simulink model "GripTask"  (R2022b)
settings: Solver=FixedStepDiscrete  StartTime=0.0  StopTime=Inf  FixedStep=0.001  RelTol=1e-3  EnableMultiTasking=on
InitFcn:
  | parambus = Simulink.Bus;
  | idx = 0;
  | 
  | idx = idx + 1;
  | parambus.Elements(idx) = Simulink.BusElement;
  | parambus.Elements(idx).Name = 'ScreenOn';
  | parambus.Elements(idx).DataType = 'uint8';
  | parambus.Elements(idx).Dimensions = [1, 1];
  | 
  | idx = idx + 1;
  | parambus.Elements(idx) = Simulink.BusElement;
  | parambus.Elements(idx).Name = 'DelayPeriod';
  | parambus.Elements(idx).DataType = 'uint16';
  | parambus.Elements(idx).Dimensions = [1, 2];
  | 
  | idx = idx + 1;
  | parambus.Elements(idx) = Simulink.BusElement;
  | parambus.Elements(idx).Name = 'TargetHoldTime';
  | parambus.Elements(idx).DataType = 'uint16';
  | parambus.Elements(idx).Dimensions = [1, 1];
  | 
  | idx = idx + 1;
  | parambus.Elements(idx) = Simulink.BusElement;
  | parambus.Elements(idx).Name = 'TargetScaling';
  | parambus.Elements(idx).DataType = 'uint8';
  | parambus.Elements(idx).Dimensions = [1, 1];
  | 
  | idx = idx + 1;
  | parambus.Elements(idx) = Simulink.BusElement;
  | parambus.Elements(idx).Name = 'TrialTimeout';
  | parambus.Elements(idx).DataType = 'uint16';
  | parambus.Elements(idx).Dimensions = [1, 1];
  | 
  | idx = idx + 1;
  | parambus.Elements(idx) = Simulink.BusElement;
  | parambus.Elements(idx).Name = 'GripCalibration';
  | parambus.Elements(idx).DataType = 'single';
  | parambus.Elements(idx).Dimensions = [1, 2];
  | 
  | idx = idx + 1;
  | parambus.Elements(idx) = Simulink.BusElement;
  | parambus.Elements(idx).Name = 'GripTarget';
  | parambus.Elements(idx).DataType = 'single';
  | parambus.Elements(idx).Dimensions = [1, 1];
  | 
  | idx = idx + 1;
  | parambus.Elements(idx) = Simulink.BusElement;
  | parambus.Elements(idx).Name = 'TaskMode';
  | parambus.Elements(idx).DataType = 'uint8';
  | parambus.Elements(idx).Dimensions = [1, 1];
  | 
  | idx = idx + 1;
  | parambus.Elements(idx) = Simulink.BusElement;
  | parambus.Elements(idx).Name = 'BuzzDuration';
  | parambus.Elements(idx).DataType = 'uint16';
  | parambus.Elements(idx).Dimensions = [1, 1];
  | 
  | FileLoggerEntry = Simulink.Bus;
  | FileLoggerEntry.Elements(1) = Simulink.BusElement;
  | FileLoggerEntry.Elements(1).Name = 'FileType';
  | FileLoggerEntry.Elements(1).DataType = 'uint8';
  | FileLoggerEntry.Elements(1).Dimensions = [1, 1];
  | FileLoggerEntry.Elements(2) = Simulink.BusElement;
  | FileLoggerEntry.Elements(2).Name = 'FieldName';
  | FileLoggerEntry.Elements(2).DataType = 'uint8';
  | FileLoggerEntry.Elements(2).Dimensions = [1, 20];
  | FileLoggerEntry.Elements(3) = Simulink.BusElement;
  | FileLoggerEntry.Elements(3).Name = 'DataType';
  | FileLoggerEntry.Elements(3).DataType = 'uint8';
  | FileLoggerEntry.Elements(3).Dimensions = [1, 6];
  | FileLoggerEntry.Elements(4) = Simulink.BusElement;
  | FileLoggerEntry.Elements(4).Name = 'NumElements';
  | FileLoggerEntry.Elements(4).DataType = 'uint8';
  | FileLoggerEntry.Elements(4).Dimensions = [1, 1];
  | FileLoggerEntry.Elements(5) = Simulink.BusElement;
  | FileLoggerEntry.Elements(5).Name = 'Data';
  | FileLoggerEntry.Elements(5).DataType = 'double';
  | FileLoggerEntry.Elements(5).Dimensions = [1, 255];
undefined symbols (not defined in the file): Ended, Single
libraries: speedgoatlib_IO191 x3, Lab_Library x2, slrealtimeseriallib x1, slrealtimeiplib x1
settings Model: Creator=irwin  LastModifiedBy=l-zirwin
settings SolverCC: ConcurrentTasks=on  AlgebraicLoopSolver=TrustRegion  PositivePriorityOrder=on  InsertRTBMode=Never (minimum delay)
settings DataIOCC: SaveFormat=Array  SaveState=on  SignalLoggingName=logsOut
settings OptimizationCC: BlockReduction=off  BooleanDataType=off  OptimizeBlockIOStorage=off  BufferReuse=off  GlobalBufferReuse=off  ExpressionFolding=off  LocalBlockOutputs=off  InitFltsAndDblsToZero=on  OptimizeDataStoreBuffers=off  BusAssignmentInplaceUpdate=off
settings DebuggingCC: SaveWithParameterizedLinksMsg=none  UnderspecifiedInitializationDetection=Classic  MergeDetectMultiDrivingBlocksExec=none  CheckExecutionContextPreStartOutputMsg=on  SignalResolutionControl=TryResolveAllWithWarning  TasksWithSamePriorityMsg=none  UnconnectedInputMsg=warning  UnconnectedOutputMsg=warning  UnconnectedLineMsg=warning  SFUnexpectedBacktrackingDiag=warning  SFNoUnconditionalDefaultTransitionDiag=warning  SFExecutionAtInitializationDiag=none  SFMachineParentedDataDiag=warning  ArithmeticOperatorsInVariantConditions=warning
settings HardwareCC: ProdBitPerLong=64  ProdLongLongMode=on  ProdHWDeviceType=Intel->x86-64 (Linux 64)
settings ModelReferenceCC: EnableRefExpFcnMdlSchedulingChecks=on  PropagateSignalLabelsOutOfModel=off
settings SFSimCC: SimUseLocalCustomCode=off  SimTargetLang=C++
settings RTWCC: Description=Simulink Real-Time  SystemTargetFile=slrealtime.tlc  TemplateMakefile=slrealtime_default_tmf  RTWUseLocalCustomCode=off  Toolchain=Simulink Real-Time Toolchain  BuildConfiguration=Faster Runs  CodeExecutionProfiling=on  TargetLang=C++  DLArmComputeVersion=19.05
settings CodeAppCC: StateflowObjectComments=on
settings SimulinkRealTimeTargetCC: MATLABClassNameForMDSCustomization=Simulink.SoftwareTarget.GRTCustomization  UseGCCFastMath=on
settings ConfigComp: CovMetricSettings=dw  CovSaveCumulativeToWorkspaceVar=on  CovSaveSingleToWorkspaceVar=on  CovExternalEMLEnable=off  CovSFcnEnable=off

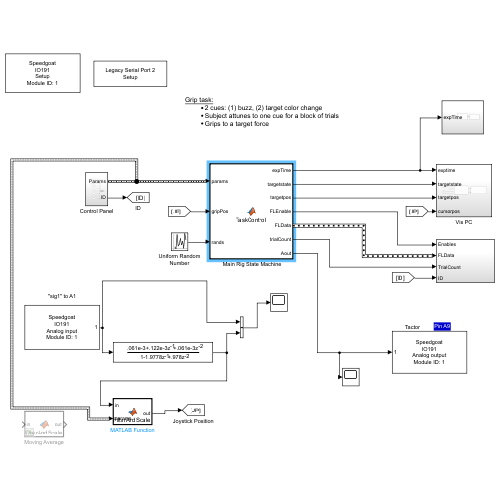
[thumbnail: Simulink's stored preview of the top-level diagram]
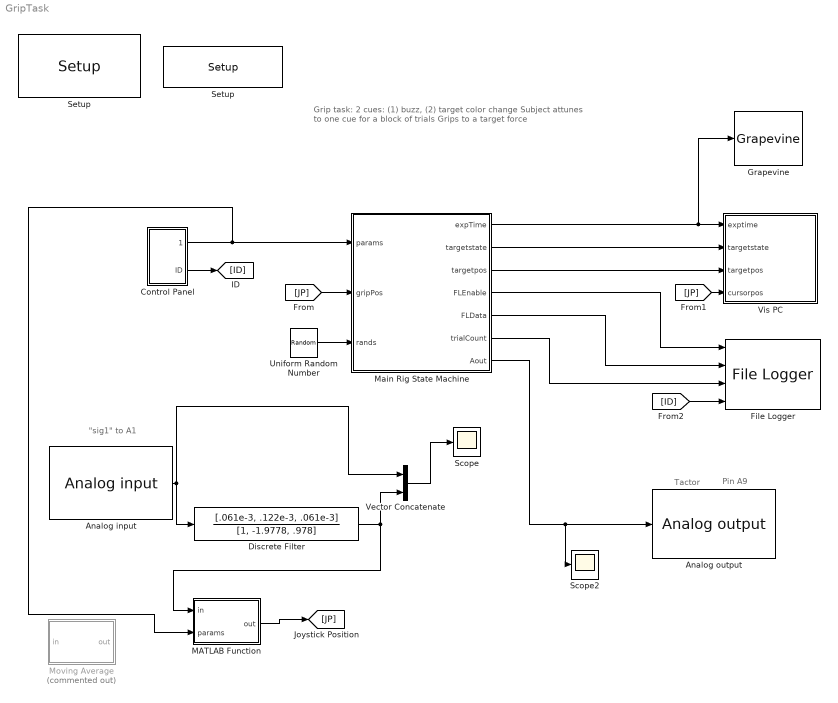
== system GripTask ==
  note: "sig1" to A1
  note: Grip task:
      | 2 cues: (1) buzz, (2) target color change
      | Subject attunes to one cue for a block of trials
      | Grips to a target force
  note: Tactor
  note: Pin A9
  " Main Rig State Machine" : MATLAB Function  TreatAsAtomicUnit=on
  "Analog input " : speedgoatlib_IO191/Analog input   parModuleId=1  parSampleTime=-1  parPciSlot=-1  parAdcChannels=1  parAdcMode=2  parAdcRanges=4  parAdcRate=100000  parAdcInitValues=[0 0]  parAdcResets=[1 1]
      settings: SourceProductName=Simulink Real-Time: Speedgoat I/O Blockset
  "Analog output " : speedgoatlib_IO191/Analog output   parModuleId=1  parSampleTime=-1  parPciSlot=-1  parDacChannels=1  parModuleType=1  parDacRanges=5  parDacInitValues=0  parDacResets=1
      settings: SourceProductName=Simulink Real-Time: Speedgoat I/O Blockset
  Control Panel : Subsystem
  Discrete Filter : DiscreteFilter  Numerator=[.061e-3, .122e-3, .061e-3]  Denominator=[1, -1.9778, .978]
  File Logger : Lab_Library/File Logger  SystemSampleTime=-1  VariantActivationTime=update diagram  Latency=0  AutoFrameSizeCalculation=off
  Grapevine : Lab_Library/Grapevine  SystemSampleTime=-1  VariantActivationTime=update diagram  Latency=0  AutoFrameSizeCalculation=off
  MATLAB Function : MATLAB Function  TreatAsAtomicUnit=on
  Moving Average : MATLAB Function  Commented=on  TreatAsAtomicUnit=on
  Scope : Scope
  Scope2 : Scope
  Setup : slrealtimeseriallib/Mainboard/Setup  port=Legacy Serial Port 2  baud=115200  width=8  nstop=1  parity=None  ctsmode=off
  "Setup " : speedgoatlib_IO191/Setup   parModuleId=1  parPciSlot=-1  parTriggerSignal=TTL  parAdcChannels=1  parAdcRanges=4  parAdcChannel1=on  parAdcChannel2=off  parAdcChannel3=off  parAdcChannel4=off  parAdcChannel5=off  parAdcChannel6=off  parAdcChannel7=off  parAdcChannel8=off  parAdcMode=Single-Ended  parAdcRate=100000  parAdcRange11=+-5.12 V  parAdcRange21=+-24.576 V  parAdcRange12=+-2.56 V  parAdcRange22=+-24.576 V  parAdcRange13=+-2.56 V  parAdcRange23=+-24.576 V  parAdcRange14=+-2.56 V  parAdcRange24=+-24.576 V  parAdcRange15=+-10.24 V  parAdcRange25=+-24.576 V  parAdcRange16=+-10.24 V  parAdcRange26=+-24.576 V  parAdcRange17=+-10.24 V  parAdcRange27=+-24.576 V  parAdcRange18=+-10.24 V  parAdcRange28=+-24.576 V  parDacChannels=1  parDacChannel1=on  parDacChannel2=off  parDacChannel3=off  parDacChannel4=off  parDacMode=Single-Ended  parDacRanges=5  parDacInitValues=0  parDacResets=1  parDacRange1=+-2.5 V  parDacInitValue1=0  parDacReset1=on  parDacRange2=+-10 V  parDacInitValue2=0  parDacReset2=on  parDacRange3=+-10 V  parDacInitValue3=0  parDacReset3=on  parDacRange4=+-10 V  parDacInitValue4=0  parDacReset4=on  parDiChannels=[1 2 3 4 5 6 7 8 9 10 11 12 13 14 15 16]  parDoChannels=zeros(1,0)  parDioFirstControl=zeros(1,0)  parDioSecondControl=0  parDioChannel1=In  parExtra1=I  parExtra2=I  parExtra3=I  parDioChannel2=In  parDioChannel3=In  parDioChannel4=In  parDioChannel5=In  parDioChannel6=In  parDioChannel7=In  parDioChannel8=In  parDioChannel9=In  parDoInitValues=[0 0 0 0]  parDoResets=[1 1 1 1]  parDoInitValue1=0  parDoReset1=on  parDoInitValue2=0  parDoReset2=on  parDoInitValue3=0  parDoReset3=on  parDoInitValue4=0  parDoReset4=on  parDoInitValue5=0  parDoReset5=on  parDoInitValue6=0  parDoReset6=on  parDoInitValue7=0  parDoReset7=on  parDoInitValue8=0  parDoReset8=on  parDoInitValue9=0  parDoReset9=on  parDoInitValue10=0  parDoReset10=on  parDoInitValue11=0  parDoReset11=on  parDoInitValue12=0  parDoReset12=on  parDoInitValue13=0  parDoReset13=on  parDoInitValue14=0  parDoReset14=on  parDoInitValue15=0  parDoReset15=on  parDoInitValue16=0  parDoReset16=on
      settings: SourceProductName=Simulink Real-Time: Speedgoat I/O Blockset
  Uniform Random Number : UniformRandomNumber  Minimum=[0, 0, 0, 0]  Maximum=[2, 2, 2, 1]  Seed=[0, 64, 71, 6]  SampleTime=.001
  Vector Concatenate : Concatenate
  Vis PC : Subsystem
  wires:
  " Main Rig State Machine"/1(expTime) -> Grapevine/1, Vis PC/1(exptime)
  " Main Rig State Machine"/2(targetstate) -> Vis PC/2(targetstate)
  " Main Rig State Machine"/4(FLEnable) -> File Logger/1
  " Main Rig State Machine"/5(FLData) -> File Logger/2
  " Main Rig State Machine"/6(trialCount) -> File Logger/3
  [JP] -> " Main Rig State Machine"/2(gripPos)
  [JP] -> Vis PC/4(cursorpos)
  Control Panel/2(ID) -> [ID]
  [ID] -> File Logger/4
  Control Panel/1(Params) -> MATLAB Function/2(params), " Main Rig State Machine"/1(params)
  Uniform Random Number/1 -> " Main Rig State Machine"/3(rands)
  " Main Rig State Machine"/3(targetpos) -> Vis PC/3(targetpos)
  "Analog input "/1 -> Vector Concatenate/1, Discrete Filter/1
  " Main Rig State Machine"/7(Aout) -> Scope2/1, "Analog output "/1
  Discrete Filter/1 -> MATLAB Function/1(in), Vector Concatenate/2
  Vector Concatenate/1 -> Scope/1
  MATLAB Function/1(out) -> [JP]

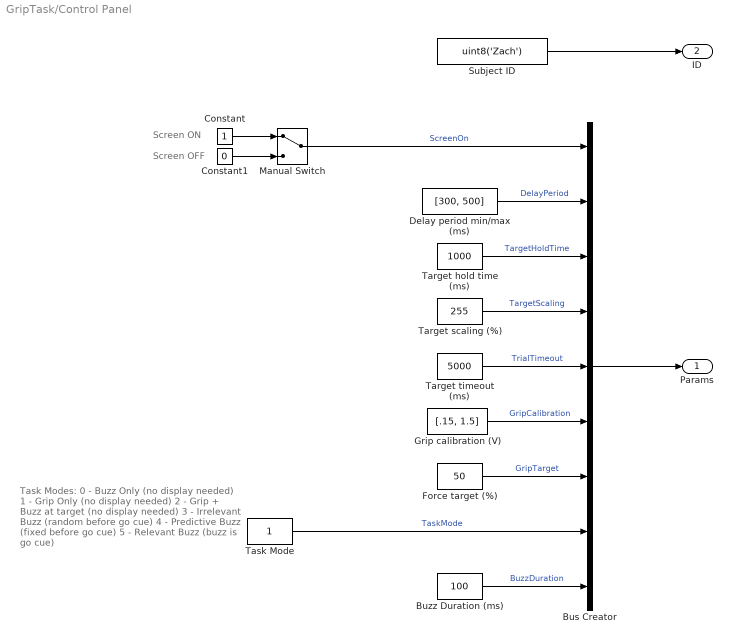
== system GripTask/Control Panel ==
  note: Task Modes:
      | 0 - Buzz Only (no display needed)
      | 1 - Grip Only (no display needed)
      | 2 - Grip + Buzz at target (no display needed)
      | 3 - Irrelevant Buzz (random before go cue)
      | 4 - Predictive Buzz (fixed before go cue)
      | 5 - Relevant Buzz (buzz is go cue)
  note: Screen ON
  note: Screen OFF
  Bus Creator : BusCreator  Inputs=9  OutDataTypeStr=Bus: parambus  NonVirtualBus=on
      settings: InheritFromInputs=off
  Buzz Duration (ms) : Constant  Value=100  OutDataTypeStr=uint16
  Constant : Constant  OutDataTypeStr=uint8
  Constant1 : Constant  Value=0  OutDataTypeStr=uint8
  Delay period min/max (ms) : Constant  Value=[300, 500]  OutDataTypeStr=uint16
  Force target (%) : Constant  Value=50  OutDataTypeStr=single
  Grip calibration (V) : Constant  Value=[.15, 1.5]  OutDataTypeStr=single
  Manual Switch : ManualSwitch
  Subject ID : Constant  Value=uint8('Zach')  OutDataTypeStr=uint8
  Target hold time (ms) : Constant  Value=1000  OutDataTypeStr=uint16
  Target scaling (%) : Constant  Value=255  OutDataTypeStr=uint8
  Target timeout (ms) : Constant  Value=5000  OutDataTypeStr=uint16
  Task Mode : Constant  OutDataTypeStr=uint8
  Params : Outport
  ID : Outport  Port=2
  wires:
  Delay period min/max (ms)/1 -> Bus Creator/2  "DelayPeriod"
  Manual Switch/1 -> Bus Creator/1  "ScreenOn"
  Constant1/1 -> Manual Switch/2
  Constant/1 -> Manual Switch/1
  Bus Creator/1 -> Params/1
  Target hold time (ms)/1 -> Bus Creator/3  "TargetHoldTime"
  Subject ID/1 -> ID/1
  Target timeout (ms)/1 -> Bus Creator/5  "TrialTimeout"
  Target scaling (%)/1 -> Bus Creator/4  "TargetScaling"
  Grip calibration (V)/1 -> Bus Creator/6  "GripCalibration"
  Force target (%)/1 -> Bus Creator/7  "GripTarget"
  Task Mode/1 -> Bus Creator/8  "TaskMode"
  Buzz Duration (ms)/1 -> Bus Creator/9  "BuzzDuration"

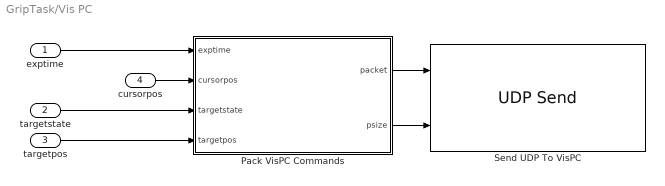
== system GripTask/Vis PC ==
  exptime : Inport
  targetstate : Inport  Port=2
  targetpos : Inport  Port=3
  cursorpos : Inport  Port=4
  Pack VisPC Commands : MATLAB Function  TreatAsAtomicUnit=on
  Send UDP To VisPC : slrealtimeiplib/UDP Send  useHostTargetConn=off  toAddress='192.168.44.2'  toPort=11114  sampleTime=-1  enableMessage=off  ipAddress='192.168.44.1'  localPort=11114
  wires:
  cursorpos/1 -> Pack VisPC Commands/2(cursorpos)
  Pack VisPC Commands/1(packet) -> Send UDP To VisPC/1
  Pack VisPC Commands/2(psize) -> Send UDP To VisPC/2
  targetstate/1 -> Pack VisPC Commands/3(targetstate)
  exptime/1 -> Pack VisPC Commands/1(exptime)
  targetpos/1 -> Pack VisPC Commands/4(targetpos)

== matlab function GripTask/Vis PC/Pack VisPC Commands ==
  data: exptime input; cursorpos input; targetstate input; packet output; psize output; targetpos input
%
% targetstate [4 x 3]: state of each target (home, narrow, wide)
%   * Row 1: Target visibility
%   * Row 2: Target hit indicators
%   * Row 3: Target sizes
%   * Row 4: Target fill indicator

% targetpos [3 x 2]: x/y position of each target (home, narrow, wide)
%   * Col 1: Left position
%   * Col 2: Top position

function [packet, psize] = CreateVisPacket(exptime, cursorpos, targetstate, targetpos)

persistent position scale color visibility fill ...
           hitcolor basecolor ...
           hometarget reachtarget_narrow reachtarget_wide cursor

if (isempty(position))

    % definitions for available objects:
    hometarget = uint8(1);
    reachtarget_narrow = uint8(2);
    reachtarget_wide = uint8(3);
    cursor = uint8(4);
    
    % definitions for available object properties:
    position = uint8(1);
    visibility = uint8(2);
    color = uint8(3);
    scale = uint8(4);
    fill = uint8(5);

    % default property values:
    hitcolor = uint8([0, 0, 255]);
    basecolor = uint8([255, 0, 0]);

end

%%% Packet structure:
%%% [experiment_time(4b), [object_id(1b), property_id(1b), property_value(xb)] ...]

% Visibility:
pvisible = [hometarget, visibility, targetstate(1,hometarget), ...
            reachtarget_narrow, visibility, targetstate(1,reachtarget_narrow), ...
            reachtarget_wide, visibility, targetstate(1,reachtarget_wide), ...
            cursor, visibility, any(targetstate(1,:))]; % cursor visible if any target is also visible, otherwise not


% Scaling:
pscaling = [hometarget, scale, targetstate(3,hometarget), ...
            reachtarget_narrow, scale, targetstate(3,reachtarget_narrow), ...
            reachtarget_wide, scale, targetstate(3,reachtarget_wide)];


% Color:
pcolor = [];
if (targetstate(2,hometarget))
    pcolor = [pcolor, hometarget, color, hitcolor];
else
    pcolor = [pcolor, hometarget, color, basecolor];
end
if (targetstate(2,reachtarget_narrow))
    pcolor = [pcolor, reachtarget_narrow, color, hitcolor];
else
    pcolor = [pcolor, reachtarget_narrow, color, basecolor];
end
if (targetstate(2,reachtarget_wide))
    pcolor = [pcolor, reachtarget_wide, color, hitcolor];
else
    pcolor = [pcolor, reachtarget_wide, color, basecolor];
end


% Fill:
pfill = [hometarget, fill, targetstate(4,hometarget), ...
            reachtarget_narrow, fill, targetstate(4,reachtarget_narrow), ...
            reachtarget_wide, fill, targetstate(4,reachtarget_wide)];


% Position:
pposition = [cursor, position, typecast([uint16(800), cursorpos], 'uint8'), ...
             hometarget, position, typecast(uint16(targetpos(hometarget,:)), 'uint8'), ...
             reachtarget_narrow, position, typecast(uint16(targetpos(reachtarget_narrow,:)), 'uint8'), ...
             reachtarget_wide, position, typecast(uint16(targetpos(reachtarget_wide,:)), 'uint8')];


% Collect into single packet, compute size, then pad to final size:
temppacket = [typecast(exptime, 'uint8'), pvisible, pscaling, pcolor, pfill, pposition];
psize = length(temppacket);
packet = [temppacket, zeros(1,1500 - psize, 'uint8')];

== matlab function GripTask/ Main Rig State Machine ==
  data: expTime output uint32 size=1; params input; gripPos input; rands input; targetstate output; targetpos output; FLEnable output; FLData output Bus: FileLoggerEntry; trialCount output; Aout output double size=1
function [expTime, targetstate, targetpos, FLEnable, FLData, trialCount, Aout] = TaskControl(params, gripPos, rands)

persistent exp_state trial_state exp_time trial_time trial_count intparams extparams...
           targpos prev_time FLStruct

if (isempty(exp_state))
    exp_state = uint8(0);           % Experiment state variable
    trial_state = uint8(0);         % Trial state variable
    exp_time = uint32(0);           % Current experiment time
    trial_time = uint32(0);         % Current trial time
    trial_count = uint16(0);        % Count of the trials in the current run
    extparams = params;             % Initialize parameters to incoming struct
    prev_time = double(-1);         % Marker for timing
    FLStruct = genFLStruct();       % Struct array for File Logger data

    intparams = struct('TaskMode', uint8(0), ...           % 6 different task modes
                       'DelayTime', uint16(0), ...          % delay period (ms)
                       'TrialSuccess', uint8(0), ...        % trial success indicator
                       'BlankTrial', uint8(0), ...          % indicator that screen was turned off
                       'TargetHit', zeros(1,3,'uint8'), ... % hit indicators for each target + home
                       'TargetFill', ones(1,3,'uint8'), ... % fill indicators for each target + home
                       'TargetVis', zeros(1,3,'uint8'), ...  % visbility indicators for each target + home
                       'BuzzDuration', uint16(0), ...      % Duration of buzz pulse
                       'PerturbDir', single(0));            % direction of perturbation for each trial

end

%%%%%%%%%%%%%%%%%%%%%%%%%%%%%%% Defines %%%%%%%%%%%%%%%%%%%%%%%%%%%%%%%%%%%

% Trial states:
tstate = struct('INIT',  uint8(0), ...
                'HOME',  uint8(1), ...
                'DELAY', uint8(2), ...
                'REACH', uint8(3), ...
                'DONE',  uint8(4), ...
                'BLANK', uint8(5));

% Trial types:
tmode = struct('BUZZONLY', uint8(0), ...
                  'GRIPONLY', uint8(1), ...
                  'GRIPBUZZ', uint8(2), ...
                  'BUZZRANDCUE', uint8(3), ...
                  'BUZZFIXEDCUE', uint8(4), ...
                  'BUZZCUE', uint8(5));


% File Logger TX enables:
fenable = struct('ZENABLE', uint8(1), ...
                 'TENABLE', uint8(2), ...
                 'MENABLE', uint8(3), ...
                 'DENABLE', uint8(4), ...
                 'NENABLE', uint8(5));

%%%%%%%%%%%%%%%%%%%%%%%%% Per-timestep updates %%%%%%%%%%%%%%%%%%%%%%%%%%%%

exp_time = exp_time + uint32(1);     % Update simulation time (1 ms per function call)
trial_time = trial_time + 1;         % Update trial time

Aout = 0;           % Initialize buzz output for this timestep

FLEnable = zeros(1,5,'uint8'); % Initialize file logger enables for this timestep

% Determine target positions and sizes:
% rectangle: [left, top, width, height]
scale = double(extparams.TargetScaling)/100;
targpos = [800-(50)/2,      900-(50),           50,      50;    % HOME
           200,                400,               200,    100;         % GOCUE
           700,                0,                200,    50*scale;];  % WIDE

% Test for hit targets:
intparams.TargetHit = uint8([0,0,0]);
for i = 1:3
    if (~params.ScreenOn || ~intparams.TargetVis(i))
        continue;
    end

    if (gripPos(1) >= targpos(i,2) && gripPos(1) <= (targpos(i,2)+targpos(i,4)))
        intparams.TargetHit(i) = uint8(1);
    else
        intparams.TargetHit(i) = uint8(0);
    end
end

%%%%%%%%%%%%%%%%%%%%%%% Stateflow switch statement %%%%%%%%%%%%%%%%%%%%%%%%

switch exp_state % Primary taskflow (experiment)
    case 0      % Initializing the File Logger
        
        %Send Z struct translator to File Logger:
        FLEnable(fenable.ZENABLE) = uint8(1);
        
        trial_state = tstate.INIT;
        exp_state = uint8(1);

    case 1      % Run the experiment
        switch trial_state % Secondary taskflow (per trial)

            case tstate.INIT

                %Pick up changes to trial parameters:
                extparams = params;
                
                % Determine the task mode for this trial:
                intparams.TaskMode = extparams.TaskMode;

                % Determine the buzz duration for this trial:
                if intparams.TaskMode == tmode.GRIPONLY
                    intparams.BuzzDuration = uint16(0);
                else
                    intparams.BuzzDuration = extparams.BuzzDuration;
                end

                % Determine delay period time:
                switch intparams.TaskMode
                    case {tmode.BUZZONLY, tmode.GRIPBUZZ, tmode.BUZZRANDCUE}
                        intparams.DelayTime = uint16(rands(4)*double(diff(extparams.DelayPeriod)) + double(extparams.DelayPeriod(1)));
                    case tmode.BUZZFIXEDCUE
                        intparams.DelayTime = uint16(mean(double(extparams.DelayPeriod)));
                    otherwise
                        intparams.DelayTime = uint16(0);
                end

                % Reset target vis info:
                intparams.TargetHit = zeros(1,3,'uint8');
                intparams.TargetVis = uint8([1, 0, 1]); % show HOME and WIDE target

                % Blank recording trial according to screen selection in Control Panel:
                intparams.BlankTrial = uint8(~extparams.ScreenOn);
                
                % Update File Logger struct with new trial params:
                FLStruct = updateFLParams(FLStruct, extparams, intparams);
                
                % Send trial parameters to File Logger:
                FLEnable(fenable.TENABLE) = uint8(1);
                
                if (intparams.BlankTrial)
                    trial_state = tstate.BLANK;
                else
                    trial_state = tstate.HOME;
                end

                trial_count = trial_count + uint16(1);
                trial_time = uint32(0);

            case tstate.HOME

                % If cursor in home target, test for complete hold:
                if intparams.TaskMode == tmode.BUZZONLY
                    holdtime = uint16(0);
                else
                    holdtime = extparams.TargetHoldTime;
                end

                if (intparams.TargetHit(1))
                    if (prev_time < 0)
                        prev_time = double(exp_time);
                    end
                    if (exp_time - prev_time >= holdtime)
                        
                        trial_time = uint32(0);
                        trial_state = tstate.DELAY;
                                       
                    end
                else
                    prev_time = double(-1);
                end
                
                % Skip to a blank trial state if requested:
                if (~params.ScreenOn)
                    intparams.BlankTrial = uint8(1);
                    trial_state = tstate.BLANK;
                end

                %Update behavior/neural File Logger structs:
                FLStruct = updateFLData(FLStruct, gripPos, Aout, [], [], exp_time);
                
                %Send measured behavior to File Logger:
                FLEnable([fenable.MENABLE]) = uint8(1);

            case tstate.DELAY

                % Test for cursor in home target and complete delay period:
                if intparams.TaskMode == tmode.BUZZONLY
                    holdtime = uint16(0);
                else
                    holdtime = extparams.TargetHoldTime;
                end

                if (intparams.TargetHit(1))
                    if (exp_time - prev_time >= holdtime + intparams.BuzzDuration + intparams.DelayTime)
%                         intparams.TargetVis(1) = uint8(0);
%                         intparams.TargetFill = uint8([1, 1, 1]);
                        prev_time = double(-1);
                        if (intparams.TaskMode == tmode.BUZZONLY)
                            trial_state = tstate.DONE;
                        else
                            trial_state = tstate.REACH;
                        end
                    end
                else
                    prev_time = double(-1);
                    trial_state = tstate.DONE;
                    intparams.TrialSuccess = uint8(0);
                end

                if intparams.TaskMode == tmode.BUZZONLY && trial_time < intparams.BuzzDuration
                    % Generate ongoing sine wave based on trial time:
                    Aout = 0.167 * sin(2*pi*100*double(trial_time)/1000);
                else
                    Aout = 0;
                end

                % Skip to a blank trial state if requested:
                if (~params.ScreenOn)
                    intparams.BlankTrial = uint8(1);
                    trial_state = tstate.BLANK;
                end

                %Update behavior/neural File Logger structs:
                FLStruct = updateFLData(FLStruct, gripPos, Aout, [], [], exp_time);
                
                %Send measured behavior + Neural to File Logger:
                FLEnable([fenable.MENABLE,fenable.NENABLE]) = uint8(1);
            
            case tstate.REACH
                
                if (intparams.TargetHit(3))
                    if (prev_time < 0)
                        prev_time = double(exp_time);
                    end
                    if (exp_time - prev_time >= extparams.TargetHoldTime)
                        prev_time = double(-1);
                        trial_state = tstate.DONE;
                        intparams.TrialSuccess = uint8(1);
                    end
                else
                    prev_time = double(-1);
                end

                if (trial_time >= extparams.TrialTimeout)
                    trial_state = tstate.DONE;
                    intparams.TrialSuccess = uint8(0);
                end

                if (trial_time <= 1000) % display go cue
                    intparams.TargetVis(2) = uint8(1);
                    intparams.TargetFill(2) = uint8(1); % Go!
                else
                    intparams.TargetVis(2) = uint8(0);
                end

                % Skip to a blank trial state if requested:
                if (~params.ScreenOn)
                    intparams.BlankTrial = uint8(1);
                    trial_state = tstate.BLANK;
                end

                %Update behavior/neural File Logger structs:
                FLStruct = updateFLData(FLStruct, gripPos, Aout, [], [], exp_time);
                
                %Send measured behavior to File Logger:
                FLEnable([fenable.MENABLE]) = uint8(1);

            case tstate.DONE

%                 Aout = single(0);

                intparams.TargetHit = zeros(1,3,'uint8');
                intparams.TargetVis = uint8([1, 0, 1]);

                if (intparams.TaskMode ~= tmode.GRIPONLY || intparams.TrialSuccess == 0)
                    trial_state = tstate.INIT;
                else
                    intparams.TargetVis(2) = uint8(1);
                    intparams.TargetFill(2) = uint8(0); % Relax
                    if (prev_time < 0)
                        prev_time = double(exp_time);
                    end
                    if (exp_time - prev_time >= 1000)
                        prev_time = double(-1);
                        trial_state = tstate.INIT;
                        intparams.TargetVis(2) = uint8(0);
                    end
                    
                end


                %Update behavior/neural File Logger structs:
                FLStruct = updateFLData(FLStruct, gripPos, Aout, [], [], exp_time);

                % Update File Logger struct with new trial params:
                FLStruct = updateFLParams(FLStruct, extparams, intparams);

                % Send trial parameters to File Logger:
                FLEnable([fenable.MENABLE, fenable.TENABLE]) = uint8(1);

            case tstate.BLANK

                Aout = 0;

                intparams.TargetHit = zeros(1,3,'uint8');
                intparams.TargetFill = ones(1,3,'uint8');
                intparams.TargetVis = zeros(1,3,'uint8');

                if (trial_time >= 20000 || params.ScreenOn)
                    trial_state = tstate.DONE;
                    intparams.TrialSuccess = uint8(0);
                end

                %Update behavior/neural File Logger structs:
                FLStruct = updateFLData(FLStruct, gripPos, Aout, [], [], exp_time);
                
                %Send measured behavior to File Logger:
                FLEnable([fenable.MENABLE]) = uint8(1);
        end
end


%%%%%%%%%%%%%%%%%%%%%%%% Assign Output Variables: %%%%%%%%%%%%%%%%%%%%%%%%%

expTime = exp_time;

FLData = FLStruct;

% targetstate = [intparams.TargetVis; intparams.TargetHit; repelem(extparams.TargetScaling,1,3); intparams.TargetFill];
targetstate = [intparams.TargetVis; intparams.TargetHit; [uint8(0), uint8(0), extparams.TargetScaling]; intparams.TargetFill];

targetpos = targpos(:,1:2);

trialCount = trial_count;

end

%%%%%%%%%%%%%%%%%%%%%%%%%%% Helper Functions: %%%%%%%%%%%%%%%%%%%%%%%%%%%%%

% Initializes an array of structures for output to the File Logger:
function flStructs = genFLStruct()

%Set up initial structure for a FileLoggerEntry struct:
tempStructs = struct('FileType', uint8(0), 'FieldName', uint8(zeros(1,20)), ...
    'DataType', uint8(zeros(1,6)), 'NumElements', uint8(0), 'Data', zeros(1,255));

%Replicate N times (#params + #behavior [meas/dec] + #neural):
flStructs = repmat(tempStructs, 1, 13);

%File types:
ftype = struct('BEHAVIOR_MEAS', uint8(2), ...
               'BEHAVIOR_DEC', uint8(3), ...
               'DATA_NEUR', uint8(4), ...
               'PARAM_START', uint8(5), ...
               'PARAM_END', uint8(6));

%Set fieldnames, file types, data types:
flStructs(1) = getStruct(ftype.PARAM_START, 'DelayTime', 'uint16', 1, []);
flStructs(2) = getStruct(ftype.PARAM_START, 'TargetHoldTime', 'uint16', 1, []);
flStructs(3) = getStruct(ftype.PARAM_START, 'TargetScaling', 'uint8', 1, []);
flStructs(4) = getStruct(ftype.PARAM_START, 'TrialTimeout', 'uint16', 1, []);
flStructs(5) = getStruct(ftype.PARAM_START, 'TaskMode', 'uint8', 1, []);
flStructs(6) = getStruct(ftype.PARAM_START, 'TargetType', 'uint8', 1, []);
flStructs(7) = getStruct(ftype.PARAM_END, 'BlankTrial', 'uint8', 1, []);
flStructs(8) = getStruct(ftype.PARAM_END, 'TrialSuccess', 'uint8', 1, []);
flStructs(9) = getStruct(ftype.BEHAVIOR_MEAS, 'gripPosition', 'single', 1, []);
flStructs(10) = getStruct(ftype.BEHAVIOR_MEAS, 'ExperimentTime', 'single', 1, []);
flStructs(11) = getStruct(ftype.BEHAVIOR_MEAS, 'BuzzOut', 'double', 1, []);
flStructs(12) = getStruct(ftype.PARAM_START, 'GripCalibration', 'single', 2, []);
flStructs(13) = getStruct(ftype.PARAM_START, 'GripTarget', 'single', 1, []);
end


% Updates the File Logger array with new parameters:
function flStructs = updateFLParams(flStruct_old, extparams, intparams)

%extparams = External, tunable parameters; intparams = Internal parameters.
%e.g. extparam1 = User-set TargetScaling, intparam1 = program-set TargetType.

flStructs = flStruct_old;
flStructs(1).Data(1:length(intparams.DelayTime))      = double(intparams.DelayTime);
flStructs(2).Data(1:length(extparams.TargetHoldTime)) = double(extparams.TargetHoldTime);
flStructs(3).Data(1:length(extparams.TargetScaling))  = double(extparams.TargetScaling);
flStructs(4).Data(1:length(extparams.TrialTimeout))   = double(extparams.TrialTimeout);
flStructs(5).Data(1:length(intparams.TaskMode))      = double(intparams.TaskMode);
flStructs(7).Data(1:length(intparams.BlankTrial))     = double(intparams.BlankTrial);
flStructs(8).Data(1:length(intparams.TrialSuccess))   = double(intparams.TrialSuccess);
flStructs(12).Data(1:length(extparams.GripCalibration))   = double(extparams.GripCalibration);
flStructs(13).Data(1:length(extparams.GripTarget))   = double(extparams.GripTarget);

end

% Updates the File Logger array with new behavior/neural data:
function flStructs = updateFLData(flStruct_old, mBehavior, Aout, dBehavior, neural, eTime)

flStructs = flStruct_old;
flStructs(9).Data(1:length(mBehavior))  = double(mBehavior);
flStructs(10).Data(1:length(eTime))     = double(eTime);
flStructs(11).Data(1:length(Aout))  = double(Aout);
end

% Helper function to create an FL struct from inputs:
function ret = getStruct(filetype,fieldname,datatype,numel,data)

ft = uint8(filetype);                                   % FileType
fn = uint8([fieldname, zeros(1,20-length(fieldname))]); % FieldName
dt = uint8([datatype, zeros(1,6-length(datatype))]);    % DataType
ne = uint8(numel);                                      % NumElements
d = double([data, zeros(1,255-length(data))]);          % Data

%Create and return structure:
ret = struct('FileType', ft, 'FieldName', fn, 'DataType', dt, 'NumElements', ne, 'Data', d);

end

== matlab function GripTask/Moving Average ==
  data: in input; out output
function out = FilterAndScale(in)

persistent buffer idx

if (isempty(buffer))
    buffer = zeros(1,20);
    idx = 0;
end

idx = 1+mod(idx, length(buffer)-1);
buffer(idx) = in;

temp = (mean(buffer) - .1)/1;
if (temp > 1)
    temp = 1;
elseif (temp < 0)
    temp = 0;
end

out = uint16(900 - 900*temp); % output: 0 force = 900/bottom of screen
                              %         full force = 0/top of screen

== matlab function GripTask/MATLAB Function ==
  data: in input; out output; params input
function out = FilterAndScale(in, params)

minval = double(params.GripCalibration(1));
maxval = double(params.GripCalibration(2));
targ = double(params.GripTarget/100);

temp = (in - minval)/((maxval-minval)*targ);
if (temp > 1)
    temp = 1;
elseif (temp < 0)
    temp = 0;
end

out = uint16(900 - 900*temp); % output: 0 force = 900/bottom of screen
                              %         full force = 0/top of screen
